simulink model "E_1_Sonido_in_delay_out"  (R2019a)
settings: Solver=VariableStepAuto  StartTime=0.0  StopTime=20.0  RelTol=1e-3  EnableMultiTasking=on
libraries: dspobslib x2
settings Model: Creator=German_Ardul  LastModifiedBy=porta
settings DataIOCC: LimitDataPoints=on  ReturnWorkspaceOutputs=off
settings OptimizationCC: LifeSpan=inf
settings DebuggingCC: UnconnectedInputMsg=none  FrameProcessingCompatibilityMsg=warning  AllowSymbolicDim=off  SFUnexpectedBacktrackingDiag=warning  SFNoUnconditionalDefaultTransitionDiag=warning  SFTransitionOutsideNaturalParentDiag=none  SFExecutionAtInitializationDiag=none  ArithmeticOperatorsInVariantConditions=warning
settings ModelReferenceCC: PropagateSignalLabelsOutOfModel=off
settings SFSimCC: SimUseLocalCustomCode=off
settings RTWCC: RTWUseLocalCustomCode=off
settings CodeAppCC: StateflowObjectComments=on
settings GRTTargetCC: TargetLangStandard=C89/C90 (ANSI)
settings ConfigComp: CovMetricSettings=dw  CovHtmlReporting=on  CovSaveCumulativeToWorkspaceVar=on  CovSaveSingleToWorkspaceVar=on  CovExternalEMLEnable=off

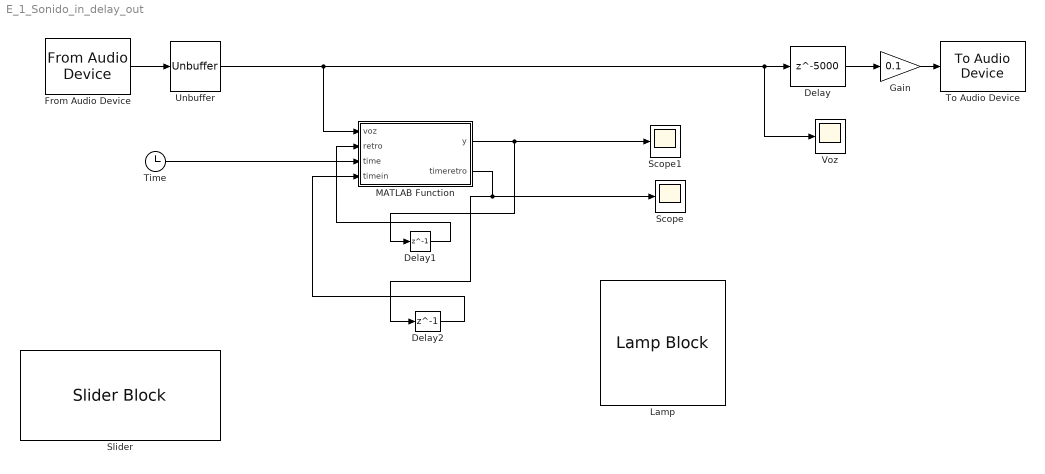
== system E_1_Sonido_in_delay_out ==
  Delay : Delay  DelayLength=5000  InputProcessing=Columns as channels (frame based)
  Delay1 : Delay  DelayLength=1  InitialCondition=0
  Delay2 : Delay  DelayLength=1  InitialCondition=0
  From Audio Device : dspobslib/From Audio Device  deviceName=Micr¾fono (HyperX Cloud Revolver S)  numChannels=1  sampleRate=44100  deviceDatatype=32-bit float  autoBufferSize=on  bufferSize=4096  queueDuration=2.0  frameSize=1024  outputDatatype=double  defaultInputChannelMapping=on  inputChannelMapping=1  outputNumOverrunSamples=off  OutputFrames=off
      settings: SourceProductName=DSP System Toolbox  SourceProductBaseCode=DS
  Gain : Gain  Gain=0.1
  Lamp : LampBlock
  MATLAB Function : MATLAB Function  TreatAsAtomicUnit=on
  Scope : Scope
  Scope1 : Scope
  Slider : SliderBlock
  Time : Clock
      settings: Decimation=20
  To Audio Device : dspobslib/To Audio Device  deviceName=Default  inheritSampleRate=on  sampleRate=44100  deviceDatatype=Determine from input data type  autoBufferSize=on  bufferSize=4096  queueDuration=1.0  defaultOutputChannelMapping=on  outputChannelMapping=1:2  outputNumUnderrunSamples=off
      settings: SourceProductName=DSP System Toolbox  SourceProductBaseCode=DS
  Unbuffer : Unbuffer
  Voz : Scope
  wires:
  From Audio Device/1 -> Unbuffer/1
  Unbuffer/1 -> MATLAB Function/1(voz), Voz/1, Delay/1
  Delay/1 -> Gain/1
  Gain/1 -> To Audio Device/1
  MATLAB Function/1(y) -> Scope1/1, Delay1/1
  Delay1/1 -> MATLAB Function/2(retro)
  Time/1 -> MATLAB Function/3(time)
  MATLAB Function/2(timeretro) -> Delay2/1, Scope/1
  Delay2/1 -> MATLAB Function/4(timein)

== matlab function E_1_Sonido_in_delay_out/MATLAB Function ==
  data: voz input; y output; retro input; time input; timeretro output; timein input
function [y, timeretro] = fcn(voz, retro, time, timein)

if time == 0
    timeretro = 0;
else
    timeretro = timein;
end
   

if (timeretro == 0 && voz >= 0.2) || (voz >= 0.2 && time >= timeretro) 
    signal = ~logical(retro);
    y = double(signal);
    timeretro = time + 0.7;
else
    signal = logical(retro);
    y = double(signal);
    timeretro = timein;
end
end
